simulink model "esperanca"  (R2024b)
settings: Solver=VariableStepAuto  StartTime=0.0  StopTime=10.0  RelTol=1e-3
libraries: aerolibasang x3, aerolibadyn x1, aerolibatmos2 x1, shared6dof x1, sharedtransform x1
settings Model: Creator=leandrosa  LastModifiedBy=leandrosa

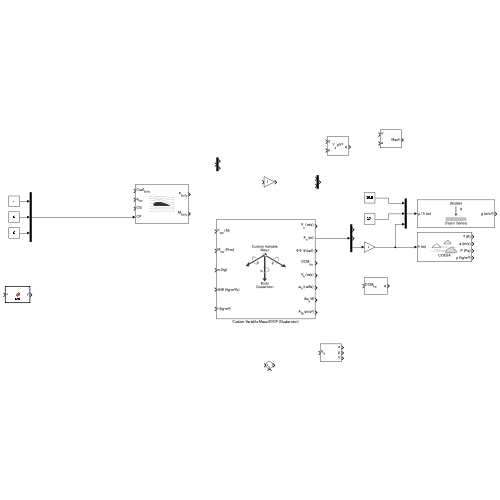
[thumbnail: Simulink's stored preview of the top-level diagram]
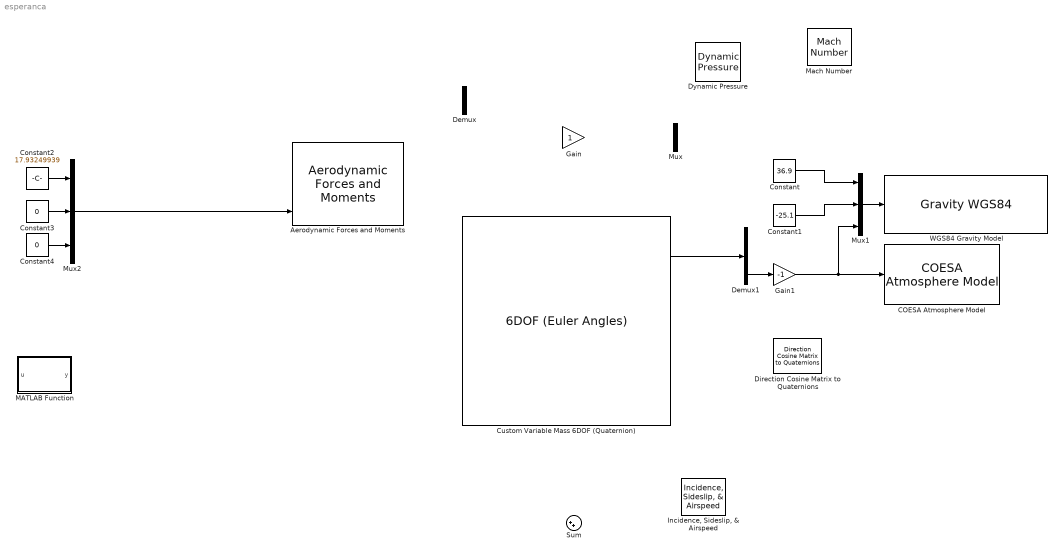
== system esperanca ==
  "Aerodynamic Forces and Moments " : aerolibadyn/Aerodynamic Forces and Moments   inputAxes=Body  outputForceAxes=Body  outputMomentAxes=Body  S=1  b=1  cbar=1
  COESA Atmosphere Model : aerolibatmos2/COESA Atmosphere Model  units=Metric (MKS)  spec=1976 COESA-extended U.S. Standard Atmosphere  model=Profile  profile_var=High temperature  profile_percent=1%  profile_alt=5 km (16404 ft)  envelope_var=High temperature  envelope_percent=1%  action=Warning
  Constant : Constant  Value=36.9
  Constant1 : Constant  Value=-25.1
  Constant2 : Constant  Value=17.93249939
  Constant3 : Constant  Value=0
  Constant4 : Constant  Value=0
  Custom Variable Mass 6DOF (Quaternion) : shared6dof/6DOF (Euler Angles)  units=Metric (MKS)  mtype=Custom Variable  rep=Quaternion  xme_0=[0 0 0]  Vm_0=[0 0 0]  eul_0=[0 0 0]  pm_0=[0 0 0]  mass_0=1.0  mass_e=0.5  mass_f=2.0  inertia=eye(3)  inertia_e=eye(3)  inertia_f=2*eye(3)  k_quat=1.0  vre_flag=off  abi_flag=off  aMode=0  xme_statename=''  Vm_statename=''  eul_statename=''  quat_statename=''  pm_statename=''  mass_statename=''
      settings: LibrarySourceBlock=aerolib6dof2/Custom Variable Mass 6DOF (Quaternion)
  Demux : Demux  Outputs=2
  Demux1 : Demux  Outputs=3
  Direction Cosine Matrix to Quaternions : sharedtransform/Direction Cosine Matrix  to Quaternions  aMode=0  action=None  tolerance=eps(2)
      settings: LibrarySourceBlock=|
      | aerolibtransform2/Direction Cosine Matrix
      | to Quaternions
  Dynamic Pressure : aerolibasang/Dynamic Pressure
  Gain : Gain
  Gain1 : Gain  Gain=-1
  "Incidence, Sideslip, & Airspeed" : aerolibasang/Incidence, Sideslip, & Airspeed
  MATLAB Function : MATLAB Function  TreatAsAtomicUnit=on
  Mach Number : aerolibasang/Mach Number
  Mux : Mux  Inputs=2
  Mux1 : Mux  Inputs=3
  Mux2 : Mux  Inputs=3
  Sum : Sum  Inputs=|++
  "WGS84 Gravity Model  " : GravityWGS84
  wires:
  Custom Variable Mass 6DOF (Quaternion)/2 -> Demux1/1
  Demux1/3 -> Gain1/1
  Gain1/1 -> Mux1/3, COESA Atmosphere Model/1
  Mux1/1 -> "WGS84 Gravity Model  "/1
  Constant/1 -> Mux1/1
  Constant1/1 -> Mux1/2
  Constant4/1 -> Mux2/3
  Constant3/1 -> Mux2/2
  Constant2/1 -> Mux2/1
  Mux2/1 -> "Aerodynamic Forces and Moments "/4

== matlab function esperanca/MATLAB Function ==
  data: u input; y output
function y = fcn(u)

y = u;
